simulink model "DiagramArticulatedSimulink"  (R2019b)
settings: Solver=ode45  StartTime=0.0  StopTime=10.0  MaxStep=0.1  RelTol=1e-3  EnableMultiTasking=on
settings Model: Creator=andre  LastModifiedBy=asmendes
settings DataIOCC: LimitDataPoints=on  SaveFormat=Array  ReturnWorkspaceOutputs=off
settings OptimizationCC: LifeSpan=inf
settings DebuggingCC: UnderspecifiedInitializationDetection=Classic  MergeDetectMultiDrivingBlocksExec=none  SolverPrmCheckMsg=warning  StateNameClashWarn=warning  SFUnexpectedBacktrackingDiag=warning  SFNoUnconditionalDefaultTransitionDiag=warning  SFExecutionAtInitializationDiag=none  ArithmeticOperatorsInVariantConditions=warning
settings HardwareCC: ProdBitPerPointer=32  ProdBitPerSizeT=32  ProdBitPerPtrDiffT=32  ProdLargestAtomicFloat=None  ProdIntDivRoundTo=Undefined  ProdEndianess=Unspecified  ProdWordSize=32  ProdHWDeviceType=32-bit Generic
settings ModelReferenceCC: PropagateSignalLabelsOutOfModel=off
settings SFSimCC: SimUseLocalCustomCode=off  CustomCodeUndefinedFunction=UseInterfaceOnly
settings RTWCC: RTWUseLocalCustomCode=off
settings CodeAppCC: StateflowObjectComments=on
settings GRTTargetCC: TargetLangStandard=C89/C90 (ANSI)  GeneratePreprocessorConditionals=Disable all
settings ConfigComp: CovMetricSettings=dw  CovHtmlReporting=on  CovSaveCumulativeToWorkspaceVar=on  CovSaveSingleToWorkspaceVar=on  CovExternalEMLEnable=off

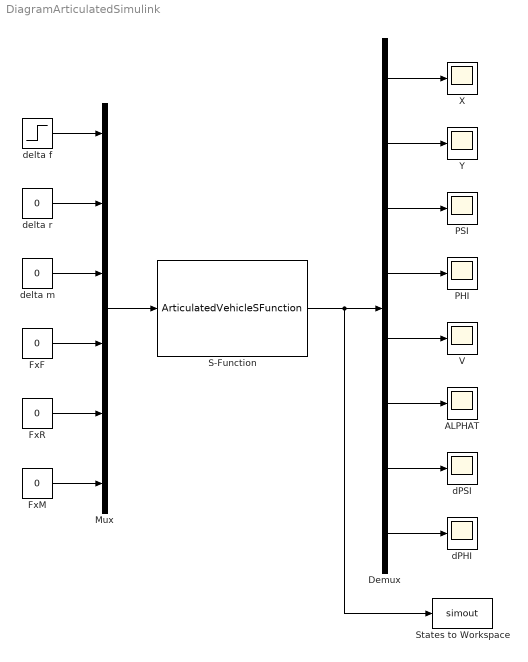
== system DiagramArticulatedSimulink ==
  ALPHAT : Scope
  Demux : Demux  Outputs=8
  FxF : Constant  Value=0
  FxM : Constant  Value=0
  FxR : Constant  Value=0
  Mux : Mux  Inputs=6
  PHI : Scope
  PSI : Scope
  S-Function : S-Function  FunctionName=ArticulatedVehicleSFunction  SFunctionDeploymentMode=off  EnableBusSupport=off
  States to Workspace : ToWorkspace  VariableName=simout  SaveFormat=Timeseries  SampleTime=-1
  V : Scope
  X : Scope
  Y : Scope
  dPHI : Scope
  dPSI : Scope
  delta f : Step  After=3*pi/180  SampleTime=0
  delta m : Constant  Value=0
  delta r : Constant  Value=0
  wires:
  delta f/1 -> Mux/1
  FxF/1 -> Mux/4
  FxR/1 -> Mux/5
  Mux/1 -> S-Function/1
  S-Function/1 -> Demux/1, States to Workspace/1
  Demux/1 -> X/1
  Demux/2 -> Y/1
  Demux/3 -> PSI/1
  Demux/4 -> PHI/1
  Demux/5 -> V/1
  Demux/6 -> ALPHAT/1
  FxM/1 -> Mux/6
  Demux/7 -> dPSI/1
  Demux/8 -> dPHI/1
  delta r/1 -> Mux/2
  delta m/1 -> Mux/3
